simulink model "runnable_1"  (R2023b)
settings: Solver=FixedStepDiscrete  StartTime=0.0  StopTime=10.0  FixedStep=0.01  RelTol=1e-3
settings Model: Creator=developer  LastModifiedBy=thabok
settings OptimizationCC: DefaultParameterBehavior=Inlined  EnhancedBackFolding=on  PassReuseOutputArgsAs=Individual arguments  ZeroExternalMemoryAtStartup=off  ZeroInternalMemoryAtStartup=off  OptimizeBlockOrder=speed  DifferentSizesBufferReuse=on  OptimizationCustomize=off  EfficientTunableParamExpr=on
settings DebuggingCC: ParameterTunabilityLossMsg=error
settings ModelReferenceCC: ModelReferenceNumInstancesAllowed=Single
settings SFSimCC: MATLABDynamicMemAlloc=off
settings RTWCC: Description=Embedded Coder  SystemTargetFile=ert.tlc  GenCodeOnly=on  TemplateMakefile=ert_default_tmf
settings CodeAppCC: ForceParamTrailComments=on  IgnoreCustomStorageClasses=off  OperatorAnnotations=on  SimulinkDataObjDesc=on  SFDataObjDesc=on  InsertBlockDesc=on
settings ERTTargetCC: TargetLangStandard=C99 (ISO)  GenerateSampleERTMain=on  SupportAbsoluteTime=off  SupportNonFinite=off  SupportComplex=off  InlinedParameterPlacement=NonHierarchical  ERTCustomFileTemplate=example_file_process.tlc

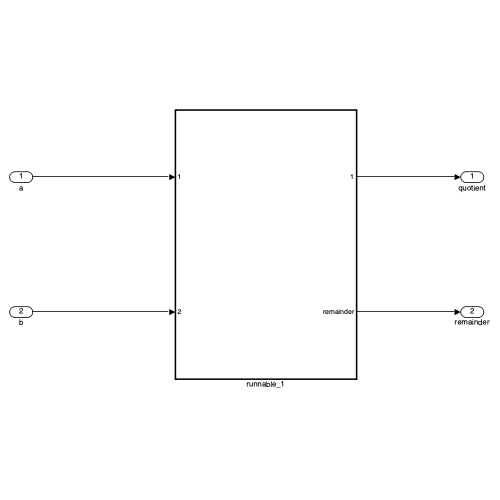
[thumbnail: Simulink's stored preview of the top-level diagram]
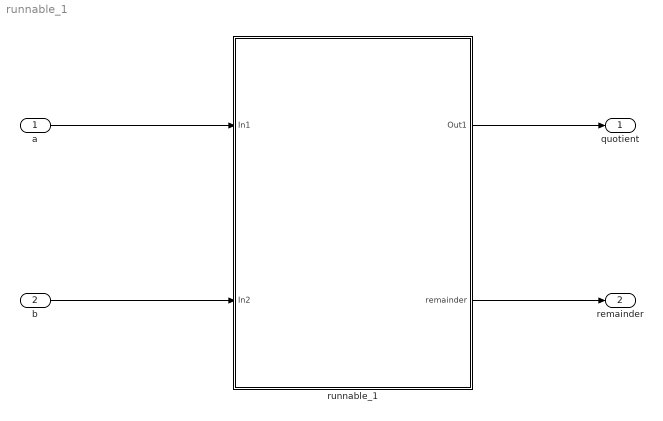
== system runnable_1 ==
  a : Inport
  b : Inport  Port=2
  runnable_1 : Subsystem  TreatAsAtomicUnit=on
      settings: RTWSystemCode=Nonreusable function  RTWFcnNameOpts=Use subsystem name
  quotient : Outport
  remainder : Outport  Port=2
  wires:
  a/1 -> runnable_1/1(In1)
  b/1 -> runnable_1/2(In2)
  runnable_1/1(Out1) -> quotient/1
  runnable_1/2(remainder) -> remainder/1

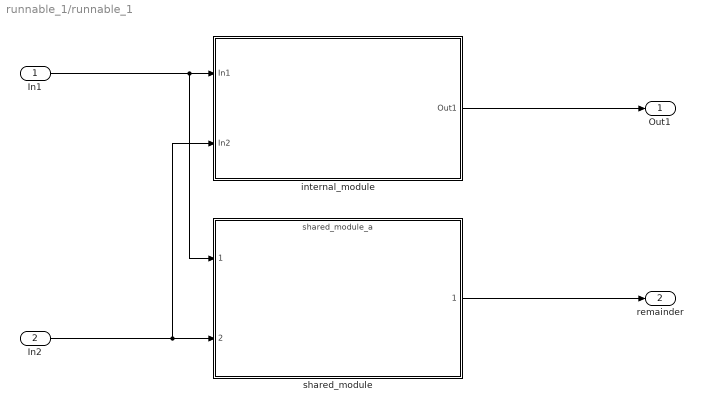
== system runnable_1/runnable_1 ==
  In1 : Inport
  In2 : Inport  Port=2
  internal_module : Subsystem
  shared_module : ModelReference  ModelNameDialog=shared_module_a.slx  SimulationMode=Normal  ModelReferenceVersion=1.10
  Out1 : Outport
  remainder : Outport  Port=2
  wires:
  In1/1 -> internal_module/1(In1), shared_module/1
  shared_module/1 -> remainder/1
  internal_module/1(Out1) -> Out1/1
  In2/1 -> internal_module/2(In2), shared_module/2

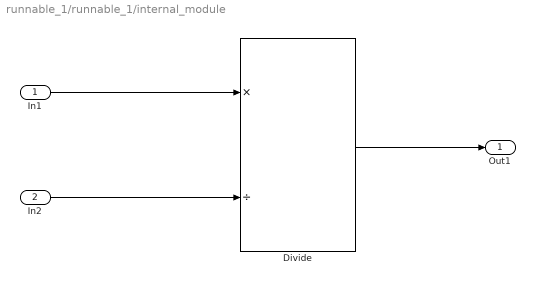
== system runnable_1/runnable_1/internal_module ==
  In1 : Inport
  In2 : Inport  Port=2
  Divide : Product  Inputs=*/
  Out1 : Outport
  wires:
  In1/1 -> Divide/1
  In2/1 -> Divide/2
  Divide/1 -> Out1/1
